simulink model "se3_2019a"  (R2019a)
settings: Solver=FixedStepAuto  StartTime=0.0  StopTime=10  FixedStep=0.005  RelTol=1e-3
settings Model: Creator=isxie  LastModifiedBy=isxie

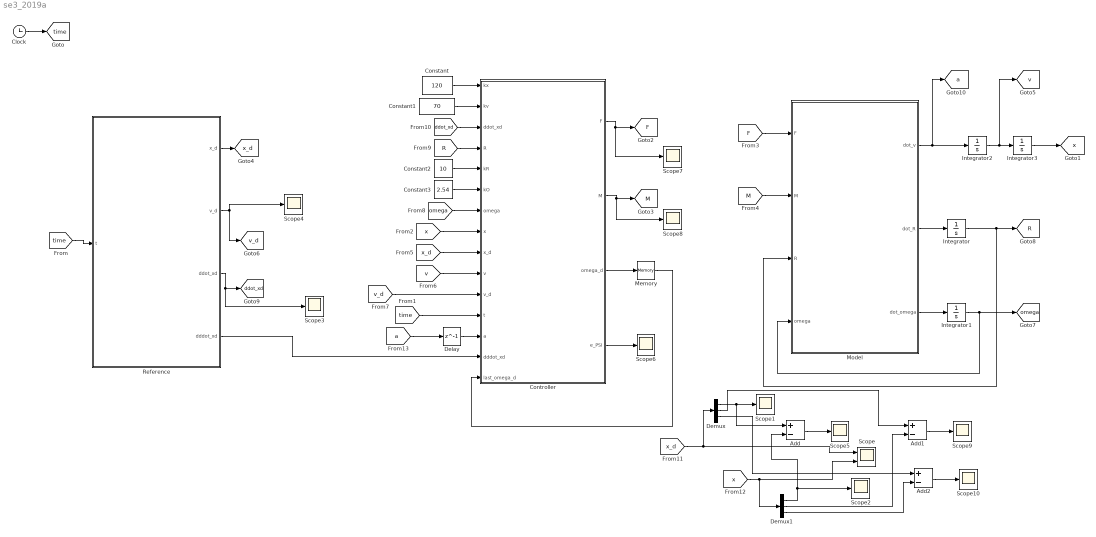
== system se3_2019a ==
  Add : Sum  Inputs=+-
  Add1 : Sum  Inputs=+-
  Add2 : Sum  Inputs=+-
  Clock : Clock
  Constant : Constant  Value=120
  Constant1 : Constant  Value=70
  Constant2 : Constant  Value=10
  Constant3 : Constant  Value=2.54
  Controller : MATLAB Function  TreatAsAtomicUnit=on
  Delay : Delay  DelayLength=1  InitialCondition=0
  Demux : Demux  Outputs=3
  Demux1 : Demux  Outputs=3
  Integrator : Integrator  InitialCondition=[1,0,0;0,1,0;0,0,1]
  Integrator1 : Integrator  InitialCondition=[0;0;0]
  Integrator2 : Integrator  InitialCondition=[0;0;0]
  Integrator3 : Integrator  InitialCondition=[0;0;0]
  Memory : Memory
  Model : MATLAB Function  TreatAsAtomicUnit=on
  Reference : MATLAB Function  TreatAsAtomicUnit=on
  Scope : Scope  NumInputPorts=2
  Scope{1..10} (10 alike) : Scope
  tag scope: F=global, M=global, R=global, a=global, ddot_xd=global, omega=global, time=global, v=global, v_d=global, x=global, x_d=global
  wires:
  Clock/1 -> [time]
  [time] -> Reference/1(t)
  [time] -> Controller/12(t)
  Model/2(dot_R) -> Integrator/1
  Model/3(dot_omega) -> Integrator1/1
  Integrator1/1 -> Model/4(omega), [omega]
  Integrator/1 -> [R], Model/3(R)
  Model/1(dot_v) -> [a], Integrator2/1
  Integrator2/1 -> [v], Integrator3/1
  [x] -> Controller/8(x)
  Controller/1(F) -> Scope7/1, [F]
  Controller/2(M) -> Scope8/1, [M]
  [M] -> Model/2(M)
  [F] -> Model/1(F)
  [x_d] -> Controller/9(x_d)
  [v] -> Controller/10(v)
  [v_d] -> Controller/11(v_d)
  Constant/1 -> Controller/1(kx)
  Constant1/1 -> Controller/2(kv)
  Constant2/1 -> Controller/5(kR)
  Constant3/1 -> Controller/6(kO)
  [omega] -> Controller/7(omega)
  [R] -> Controller/4(R)
  [ddot_xd] -> Controller/3(ddot_xd)
  Integrator3/1 -> [x]
  [x_d] -> Demux/1, Scope/1
  [x] -> Demux1/1, Scope/2
  Demux/1 -> Add/1, Scope1/1
  Demux1/1 -> Add/2, Scope2/1
  Reference/1(x_d) -> [x_d]
  Reference/3(ddot_xd) -> Scope3/1, [ddot_xd]
  Reference/2(v_d) -> [v_d], Scope4/1
  Add/1 -> Scope5/1
  [a] -> Delay/1
  Reference/4(dddot_xd) -> Controller/14(dddot_xd)
  Delay/1 -> Controller/13(a)
  Controller/3(omega_d) -> Memory/1
  Memory/1 -> Controller/15(last_omega_d)
  Controller/4(e_PSI) -> Scope6/1
  Add1/1 -> Scope9/1
  Add2/1 -> Scope10/1
  Demux/2 -> Add1/1
  Demux1/2 -> Add1/2
  Demux/3 -> Add2/1
  Demux1/3 -> Add2/2

== matlab function se3_2019a/Controller ==
  data: kx input; kv input; ddot_xd input; R input; kR input; kO input; omega input; F output; x input; x_d input; v input; v_d input; M output; t input; a input; dddot_xd input; omega_d output; last_omega_d input; e_PSI output
function [F,M,omega_d,e_PSI] = fcn(kx,kv,ddot_xd,R,kR,kO,omega,x,x_d,v,v_d,t,a,dddot_xd,last_omega_d)

m = 4.34; g = 9.8; J = diag([0.082;0.0845;0.1377]); e3 = [0;0;1];

ex = x-x_d; ev = v-v_d; ea= a-ddot_xd;

b1_d = [cos(pi*t);sin(pi*t);0];
b3_d = -(-kx*ex-kv*ev-m*g*e3+m*ddot_xd)/(norm(-kx*ex-kv*ev-m*g*e3+m*ddot_xd));
b2_d = (cross(b3_d,b1_d))/norm(cross(b3_d,b1_d));
Rd = [cross(b2_d,b3_d),b2_d,b3_d];

dot_b2_des = [-cos(pi*t)*pi;-sin(pi*t)*pi;0];
dot_f = (kx*ev + kv*ea + m*dddot_xd)/(norm(-kx*ex-kv*ev-m*g*e3+m*ddot_xd));
dot_b3 = cross(cross(b3_d,dot_f),b3_d);
mid = cross(dot_b2_des,b3_d)+cross(cross(b2_d,b3_d),dot_b3)/norm(cross(cross(b2_d,b3_d),b3_d));
dot_b1 = cross(cross(cross(b2_d,b3_d),mid),cross(b2_d,b3_d));
dot_b2 = cross(dot_b3,cross(b2_d,b3_d))+cross(b3_d,dot_b1);

dot_Rd = [dot_b1,dot_b2,dot_b3];

omega_d_mid = Rd'*dot_Rd;
omega_d = [omega_d_mid(3,2);omega_d_mid(1,3);omega_d_mid(2,1)];
dot_omega_d = (omega_d - last_omega_d)/0.005;

eR_mid = 1/2*(Rd'*R-R'*Rd);
eR = [eR_mid(3,2);eR_mid(1,3);eR_mid(2,1)];
eO = omega - R'*Rd*omega_d;

F1 = -(-kx*ex-kv*ev-m*g*e3+m*ddot_xd);
F2 = R*e3;
sk_omega = [0,-omega(3),omega(2);omega(3),0,-omega(1);-omega(2),omega(1),0];
F = dot(F1,F2);
M = -kR*eR-kO*eO+cross(omega,(J*omega))-J*(sk_omega*R'*Rd*omega_d-R'*Rd*dot_omega_d);

e_PSI = 1/2*trace(eye(3)-Rd'*R);

== matlab function se3_2019a/Reference ==
  data: t input; x_d output; v_d output; ddot_xd output; dddot_xd output
function [x_d,v_d,ddot_xd,dddot_xd]  = fcn(t)

x = 0.4*t;
y = 0.4*sin(pi*t);
z = 0.6*cos(pi*t);
d_x = 0.4;
d_y = 0.4*pi*cos(pi*t);
d_z = -0.6*pi*sin(pi*t);
dd_x = 0;
dd_y = -0.4*pi*pi*sin(pi*t);
dd_z = -0.6*pi*pi*cos(pi*t);

ddd_x = 0;
ddd_y = -0.4*pi*pi*pi*cos(pi*t);
ddd_z = 0.6*pi^3*sin(pi*t);
x_d = [x;y;z];
v_d = [d_x;d_y;d_z];
ddot_xd = [dd_x;dd_y;dd_z];
dddot_xd = [ddd_x;ddd_y;ddd_z];

== matlab function se3_2019a/Model ==
  data: dot_v output; dot_R output; F input; M input; R input; omega input; dot_omega output
function [dot_v,dot_R,dot_omega] = fcn(F,M,R,omega)

J = diag([0.082;0.0845;0.1377]); m = 4.34; e3 = [0;0;1]; g = 9.8;

sk = [0,-omega(3),omega(2);omega(3),0,-omega(1);-omega(2),omega(1),0];
dot_v = g*e3-1/m*F*R*e3;
dot_R = R*sk;
dot_omega = inv(J)*(-sk*(J*omega)+M);
